simulink subsystem "SiDLEngine"  (R2023b)
settings: Solver=VariableStepAuto  StartTime=0.0  StopTime=10.0  RelTol=1e-3
undefined symbols (not defined in the file): EnvAbsPrs, EnvAirTemp, EnvRair, PlntEngAfrStoich, PlntEngCps, PlntEngGasLhv, PlntEngInTrqLdBpt, PlntEngInTrqSpdBpt, PlntEngNeuralODE, PlntEngSAOpt, PlntEngSIDLNCyl, PlntEngSIDLTimeCETC, PlntEngSIDLTimeCVGT, PlntEngSIDLVd, PlntEngSinj, PlntEngTimeCEGR, PlntEngTimeCIRL, PlntEngTimeCIVL, PlntEngTimeCVCR, PlntEngTimeCWVA
libraries: autolibutils x2, autolibpowerinfoutils x2, autolibhevctrlrcommon x1
settings Model: ModifiedByFormat=The MathWorks, Inc.  Creator=The MathWorks, Inc.  LastModifiedBy=The MathWorks, Inc.
settings SolverCC: MaxZcPerStep=1
settings OptimizationCC: ReuseModelBlockBuffer=off
settings DebuggingCC: UnconnectedInputMsg=warning  UnconnectedOutputMsg=warning  UnconnectedLineMsg=warning
settings ModelReferenceCC: EnableRefExpFcnMdlSchedulingChecks=on
settings RTWCC: DLArmComputeVersion=19.05

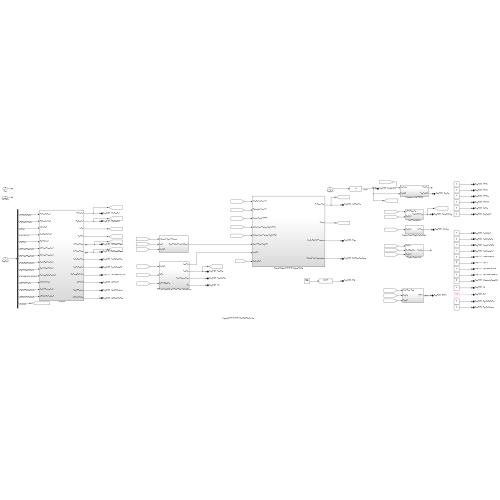
[thumbnail: Simulink's stored preview of the top-level diagram]
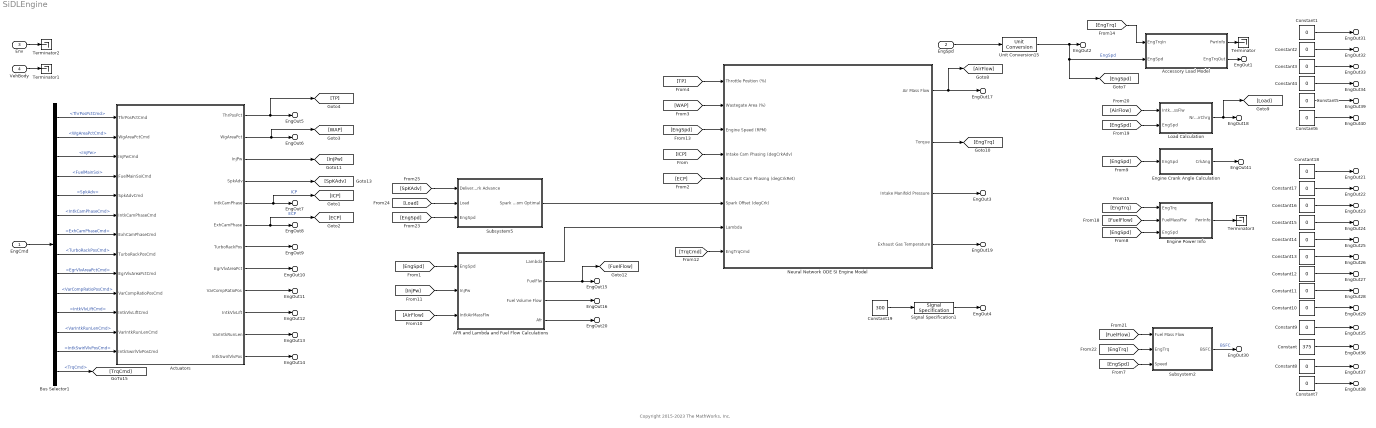
== system SiDLEngine ==
  note: Copyright 2015-2023 The MathWorks, Inc.
  EngCmd : Inport
  EngSpd : Inport  Port=2  Unit=rad/sec
  Env : Inport  Port=3
  VehBody : Inport  Port=4
  AFR and Lambda and Fuel Flow Calculations : Subsystem
  Accessory Load Model : Subsystem
  Actuators : Subsystem
  Bus Selector1 : BusSelector  OutputSignals=ThrPosPctCmd,WgAreaPctCmd,InjPw,FuelMainSoi,SpkAdv,IntkCamPhaseCmd,ExhCamPhaseCmd,TurboRackPosCmd,EgrVlvAreaPctCmd,VarCompRatioPosCmd,IntkVlvLiftCmd,VarIntkRunLenCmd,IntkSwirlVlvPosCmd,TrqCmd
  Constant : Constant  Value=375  SampleTime=-1
  Constant{1..18} (18 alike) : Constant  Value=0  SampleTime=-1
  Constant19 : Constant  Value=300
  Engine Crank Angle Calculation : Subsystem
  Engine Power Info : Subsystem
  Load Calculation : Subsystem
  Neural Network ODE SI Engine Model : Subsystem
  Signal Specification1 : SignalSpecification  Unit=K
  Subsystem2 : Subsystem
  Subsystem5 : Subsystem
  Terminator{,1..3} (4 alike) : Terminator
  Unit Conversion15 : UnitConversion
  EngOut2 : Outport  PortName=EngFdbk  Element=EngSpdOut
  EngOut5 : Outport  PortName=EngFdbk  Element=ThrPosPct
  EngOut6 : Outport  PortName=EngFdbk  Element=WgAreaPct
  EngOut7 : Outport  PortName=EngFdbk  Element=IntkCamPhase
  EngOut8 : Outport  PortName=EngFdbk  Element=ExhCamPhase
  EngOut9 : Outport  PortName=EngFdbk  Element=TurboRackPos
  EngOut10 : Outport  PortName=EngFdbk  Element=EgrVlvAreaPct
  EngOut11 : Outport  PortName=EngFdbk  Element=VarCompRatioPos
  EngOut12 : Outport  PortName=EngFdbk  Element=IntkVlvLift
  EngOut13 : Outport  PortName=EngFdbk  Element=VarIntkRunLen
  EngOut14 : Outport  PortName=EngFdbk  Element=IntkSwirlVlvPos
  EngOut3 : Outport  PortName=EngFdbk  Element=Map
  EngOut4 : Outport  PortName=EngFdbk  Element=Mat
  EngOut15 : Outport  PortName=EngFdbk  Element=FuelFlw
  EngOut16 : Outport  PortName=EngFdbk  Element=FuelVolFlw
  EngOut20 : Outport  PortName=EngFdbk  Element=Afr
  EngOut19 : Outport  PortName=EngFdbk  Element=ExhManGasTemp
  EngOut17 : Outport  PortName=EngFdbk  Element=IntkPortFlw
  EngOut1 : Outport  PortName=EngFdbk  Element=EngTrq
  EngOut18 : Outport  PortName=EngFdbk  Element=NormAirChrg
  EngOut41 : Outport  PortName=EngFdbk  Element=CrkAng
  EngOut30 : Outport  PortName=EngFdbk  Element=BSFC
  EngOut31 : Outport  PortName=EngFdbk  Element=TPHC
  EngOut32 : Outport  PortName=EngFdbk  Element=TPCO
  EngOut33 : Outport  PortName=EngFdbk  Element=TPNOx
  EngOut34 : Outport  PortName=EngFdbk  Element=TPCO2
  EngOut39 : Outport  PortName=EngFdbk  Element=CylPrs
  EngOut40 : Outport  PortName=EngFdbk  Element=EngTrqCrk
  EngOut21 : Outport  PortName=EngFdbk  Element=TurboSpd
  EngOut22 : Outport  PortName=EngFdbk  Element=TurbPrsRatio
  EngOut23 : Outport  PortName=EngFdbk  Element=CompPrsRatio
  EngOut24 : Outport  PortName=EngFdbk  Element=TurbTempOut
  EngOut25 : Outport  PortName=EngFdbk  Element=CompTempOut
  EngOut26 : Outport  PortName=EngFdbk  Element=EgrPct
  EngOut27 : Outport  PortName=EngFdbk  Element=EgrMassFlwRate
  EngOut28 : Outport  PortName=EngFdbk  Element=EgrCoolerTempOut
  EngOut29 : Outport  PortName=EngFdbk  Element=IntercoolerTempOut
  EngOut35 : Outport  PortName=EngFdbk  Element=Iat
  EngOut36 : Outport  PortName=EngFdbk  Element=Ect
  EngOut37 : Outport  PortName=EngFdbk  Element=EgrVlvDeltaPrs
  EngOut38 : Outport  PortName=EngFdbk  Element=EgrVlvInTemp
  wires:
  Actuators/11(VarIntkRunLen) -> EngOut13/1
  Constant12/1 -> EngOut27/1
  Actuators/7(TurboRackPos) -> EngOut9/1
  Actuators/6(ExhCamPhase) -> [ECP], EngOut8/1  "ECP"
  Actuators/9(VarCompRatioPos) -> EngOut11/1
  Constant1/1 -> EngOut31/1
  Engine Crank Angle Calculation/1(CrkAng) -> EngOut41/1
  [EngSpd] -> Engine Crank Angle Calculation/1(EngSpd)
  [EngSpd] -> Engine Power Info/3(EngSpd)
  Subsystem5/1(Spark Retard From Optimal) -> Neural Network ODE SI Engine Model/6(Spark Offset (degCrk))
  Accessory Load Model/2(EngTrqOut) -> EngOut1/1
  [TP] -> Neural Network ODE SI Engine Model/1(Throttle Position (%))
  [ECP] -> Neural Network ODE SI Engine Model/5(Exhaust Cam Phasing (degCrkRet))
  [FuelFlow] -> Engine Power Info/2(FuelMassFlw)
  [EngSpd] -> Neural Network ODE SI Engine Model/3(Engine Speed (RPM))
  Neural Network ODE SI Engine Model/2(Torque) -> [EngTrq]
  [ICP] -> Neural Network ODE SI Engine Model/4(Intake Cam Phasing (degCrkAdv))
  Constant13/1 -> EngOut26/1
  [EngTrq] -> Subsystem2/2(EngTrq)
  Accessory Load Model/1(PwrInfo) -> Terminator/1
  Constant/1 -> EngOut36/1
  Constant10/1 -> EngOut29/1
  Actuators/5(IntkCamPhase) -> [ICP], EngOut7/1  "ICP"
  Neural Network ODE SI Engine Model/3(Intake Manifold Pressure) -> EngOut3/1
  [InjPw] -> AFR and Lambda and Fuel Flow Calculations/2(InjPw)
  Constant8/1 -> EngOut37/1
  Constant4/1 -> EngOut34/1
  Constant15/1 -> EngOut24/1
  [AirFlow] -> AFR and Lambda and Fuel Flow Calculations/3(IntkAirMassFlw)
  Subsystem2/1(BSFC) -> EngOut30/1  "BSFC"
  [EngSpd] -> AFR and Lambda and Fuel Flow Calculations/1(EngSpd)
  [TrqCmd] -> Neural Network ODE SI Engine Model/8(EngTrqCmd)
  [Load] -> Subsystem5/2(Load)
  AFR and Lambda and Fuel Flow Calculations/3(Fuel Volume Flow) -> EngOut16/1
  Actuators/8(EgrVlvAreaPct) -> EngOut10/1
  Constant19/1 -> Signal Specification1/1
  [EngTrq] -> Engine Power Info/1(EngTrq)
  Constant7/1 -> EngOut38/1
  [EngTrq] -> Accessory Load Model/1(EngTrqIn)
  AFR and Lambda and Fuel Flow Calculations/2(FuelFlw) -> [FuelFlow], EngOut15/1
  [EngSpd] -> Load Calculation/2(EngSpd)
  AFR and Lambda and Fuel Flow Calculations/1(Lambda) -> Neural Network ODE SI Engine Model/7(Lambda)
  Neural Network ODE SI Engine Model/1(Air Mass Flow) -> [AirFlow], EngOut17/1
  [AirFlow] -> Load Calculation/1(IntkAirMassFlw)
  Bus Selector1/1 -> Actuators/1(ThrPosPctCmd)  "<ThrPosPctCmd>"
  Constant14/1 -> EngOut25/1
  [EngSpd] -> Subsystem2/3(Speed)
  Constant11/1 -> EngOut28/1
  Constant17/1 -> EngOut22/1
  Actuators/2(WgAreaPct) -> [WAP], EngOut6/1
  AFR and Lambda and Fuel Flow Calculations/4(Afr) -> EngOut20/1
  Constant6/1 -> EngOut40/1
  Constant3/1 -> EngOut33/1
  Neural Network ODE SI Engine Model/4(Exhaust Gas Temperature) -> EngOut19/1
  [EngSpd] -> Subsystem5/3(EngSpd)
  Actuators/10(IntkVlvLift) -> EngOut12/1
  Actuators/4(SpkAdv) -> [SpKAdv]
  Actuators/1(ThrPosPct) -> [TP], EngOut5/1
  Constant16/1 -> EngOut23/1
  [SpKAdv] -> Subsystem5/1(Delivered Spark Advance)
  Engine Power Info/1(PwrInfo) -> Terminator3/1
  Actuators/12(IntkSwirlVlvPos) -> EngOut14/1
  Constant9/1 -> EngOut35/1
  Constant5/1 -> EngOut39/1
  [WAP] -> Neural Network ODE SI Engine Model/2(Wastegate Area (%))
  Actuators/3(InjPw) -> [InjPw]
  [FuelFlow] -> Subsystem2/1(Fuel Mass Flow)
  Constant18/1 -> EngOut21/1
  Load Calculation/1(NrmlzdAirChrg) -> [Load], EngOut18/1
  Constant2/1 -> EngOut32/1
  EngCmd/1 -> Bus Selector1/1
  Bus Selector1/12 -> Actuators/12(VarIntkRunLenCmd)  "<VarIntkRunLenCmd>"
  Bus Selector1/2 -> Actuators/2(WgAreaPctCmd)  "<WgAreaPctCmd>"
  Bus Selector1/6 -> Actuators/6(IntkCamPhaseCmd)  "<IntkCamPhaseCmd>"
  Bus Selector1/11 -> Actuators/11(IntkVlvLiftCmd)  "<IntkVlvLiftCmd>"
  Bus Selector1/3 -> Actuators/3(InjPwCmd)  "<InjPw>"
  Bus Selector1/7 -> Actuators/7(ExhCamPhaseCmd)  "<ExhCamPhaseCmd>"
  Bus Selector1/10 -> Actuators/10(VarCompRatioPosCmd)  "<VarCompRatioPosCmd>"
  Bus Selector1/9 -> Actuators/9(EgrVlvAreaPctCmd)  "<EgrVlvAreaPctCmd>"
  Bus Selector1/13 -> Actuators/13(IntkSwirlVlvPosCmd)  "<IntkSwirlVlvPosCmd>"
  Bus Selector1/14 -> [TrqCmd]  "<TrqCmd>"
  Bus Selector1/5 -> Actuators/5(SpkAdvCmd)  "<SpkAdv>"
  Bus Selector1/8 -> Actuators/8(TurboRackPosCmd)  "<TurboRackPosCmd>"
  Bus Selector1/4 -> Actuators/4(FuelMainSoiCmd)  "<FuelMainSoi>"
  EngSpd/1 -> Unit Conversion15/1
  Unit Conversion15/1 -> Accessory Load Model/2(EngSpd), [EngSpd], EngOut2/1  "EngSpd"
  VehBody/1 -> Terminator1/1
  Env/1 -> Terminator2/1
  Signal Specification1/1 -> EngOut4/1

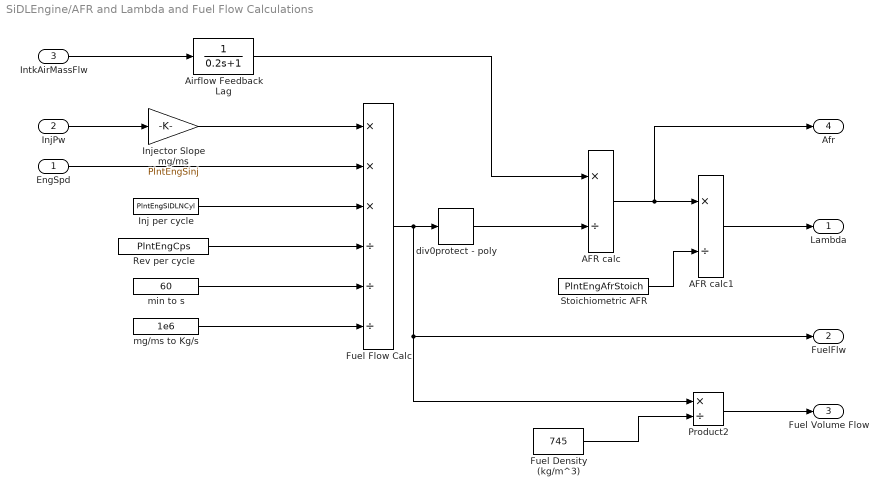
== system SiDLEngine/AFR and Lambda and Fuel Flow Calculations ==
  EngSpd : Inport
  InjPw : Inport  Port=2
  IntkAirMassFlw : Inport  Port=3
  AFR calc : Product  Inputs=*/
  AFR calc1 : Product  Inputs=*/
  Airflow Feedback Lag : TransferFcn  Denominator=[0.2 1]
  Fuel Density (kg/m^3) : Constant  Value=745
  Fuel Flow Calc : Product  Inputs=***///
  Inj per cycle : Constant  Value=PlntEngSIDLNCyl
  Injector Slope mg/ms : Gain  Gain=PlntEngSinj
  Product2 : Product  Inputs=*/
  Rev per cycle : Constant  Value=PlntEngCps
  Stoichiometric AFR : Constant  Value=PlntEngAfrStoich
  div0protect - poly : autolibutils/div0protect - poly  thresh=1e-6  ZeroCross1=off  aMode=aMode
  mg/ms to Kg/s : Constant  Value=1e6
  min to s : Constant  Value=60
  Lambda : Outport  VectorParamsAs1DForOutWhenUnconnected=off
  FuelFlw : Outport  Port=2  VectorParamsAs1DForOutWhenUnconnected=off
  Fuel Volume Flow : Outport  Port=3
  Afr : Outport  Port=4  VectorParamsAs1DForOutWhenUnconnected=off
  wires:
  Fuel Flow Calc/1 -> div0protect - poly/1, Product2/1, FuelFlw/1
  Fuel Density (kg/m^3)/1 -> Product2/2
  Product2/1 -> Fuel Volume Flow/1
  AFR calc1/1 -> Lambda/1
  IntkAirMassFlw/1 -> Airflow Feedback Lag/1
  EngSpd/1 -> Fuel Flow Calc/2
  Inj per cycle/1 -> Fuel Flow Calc/3
  Injector Slope mg/ms/1 -> Fuel Flow Calc/1
  mg/ms to Kg/s/1 -> Fuel Flow Calc/6
  min to s/1 -> Fuel Flow Calc/5
  Stoichiometric AFR/1 -> AFR calc1/2
  div0protect - poly/1 -> AFR calc/2
  InjPw/1 -> Injector Slope mg/ms/1
  AFR calc/1 -> AFR calc1/1, Afr/1
  Rev per cycle/1 -> Fuel Flow Calc/4
  Airflow Feedback Lag/1 -> AFR calc/1

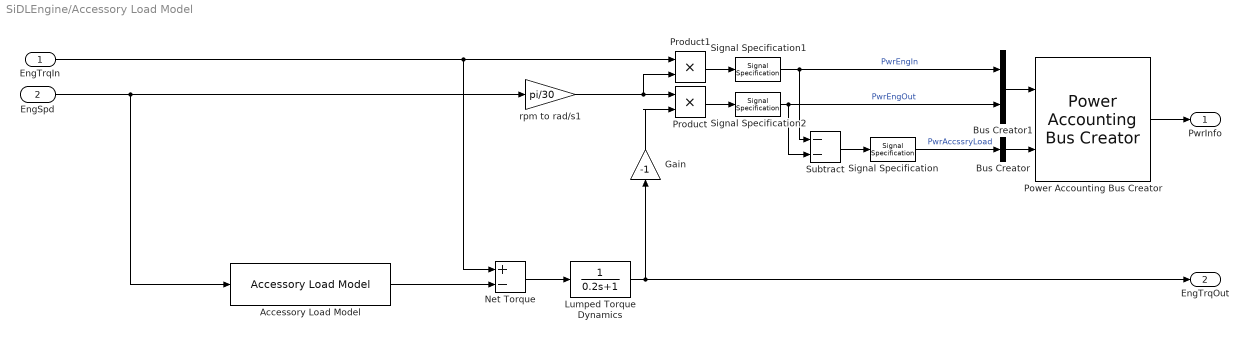
== system SiDLEngine/Accessory Load Model ==
  EngTrqIn : Inport
  EngSpd : Inport  Port=2
  Accessory Load Model : autolibhevctrlrcommon/Accessory Load Model  AccPwrTbl=PlntEngSIDLAccPwrTbl  AccSpdBpts=PlntEngSIDLAccSpdBpt
  Bus Creator : BusCreator  Inputs=1
  Bus Creator1 : BusCreator  Inputs=2
  Gain : Gain  Gain=-1
  Lumped Torque Dynamics : TransferFcn  Denominator=[0.2 1]
  Net Torque : Sum  Inputs=+-
  Power Accounting Bus Creator : autolibpowerinfoutils/Power Accounting Bus Creator  AssctBlkSelPopup=Parent  RefBlkName='libraryname/blkname'  PwrTrnsfrdCheckBox=on  PwrNotTrnsfrdCheckBox=on  PwrStoredCheckBox=off  aMode=aMode
  Product : Product
  Product1 : Product
  Signal Specification : SignalSpecification  Unit=W
  Signal Specification1 : SignalSpecification  Unit=W
  Signal Specification2 : SignalSpecification  Unit=W
  Subtract : Sum  Inputs=--
  rpm to rad/s1 : Gain  Gain=pi/30
  PwrInfo : Outport  VectorParamsAs1DForOutWhenUnconnected=off
  EngTrqOut : Outport  Port=2  Unit=N*m  VectorParamsAs1DForOutWhenUnconnected=off
  wires:
  Gain/1 -> Product/2
  Signal Specification2/1 -> Bus Creator1/2, Subtract/2  "PwrEngOut"
  Signal Specification1/1 -> Bus Creator1/1, Subtract/1  "PwrEngIn"
  rpm to rad/s1/1 -> Product/1, Product1/2
  Product1/1 -> Signal Specification1/1
  Product/1 -> Signal Specification2/1
  Power Accounting Bus Creator/1 -> PwrInfo/1
  Signal Specification/1 -> Bus Creator/1  "PwrAccssryLoad"
  Subtract/1 -> Signal Specification/1
  EngTrqIn/1 -> Net Torque/1, Product1/1
  Bus Creator1/1 -> Power Accounting Bus Creator/1
  Bus Creator/1 -> Power Accounting Bus Creator/2
  Net Torque/1 -> Lumped Torque Dynamics/1
  Lumped Torque Dynamics/1 -> Gain/1, EngTrqOut/1
  EngSpd/1 -> rpm to rad/s1/1, Accessory Load Model/1
  Accessory Load Model/1 -> Net Torque/2

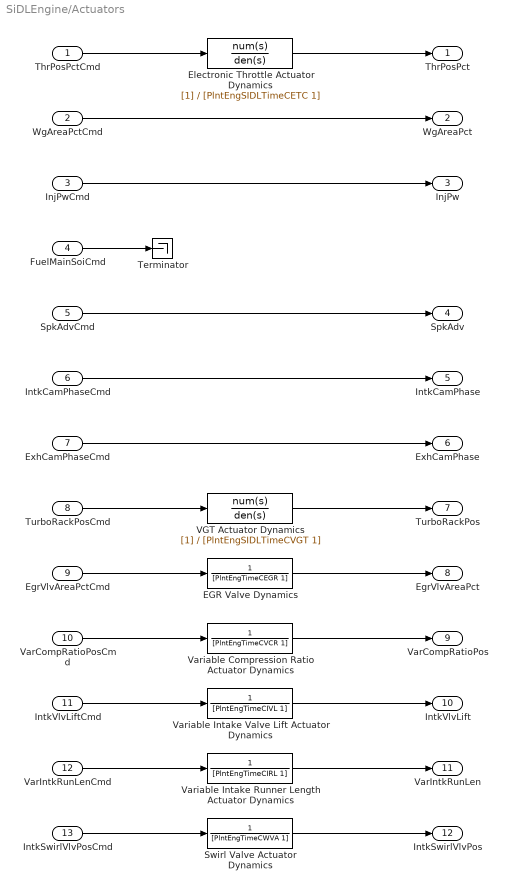
== system SiDLEngine/Actuators ==
  ThrPosPctCmd : Inport  Unit=%
  WgAreaPctCmd : Inport  Port=2  Unit=%
  InjPwCmd : Inport  Port=3  Unit=ms
  FuelMainSoiCmd : Inport  Port=4  Unit=deg
  SpkAdvCmd : Inport  Port=5  Unit=deg
  IntkCamPhaseCmd : Inport  Port=6  Unit=deg
  ExhCamPhaseCmd : Inport  Port=7  Unit=deg
  TurboRackPosCmd : Inport  Port=8  Unit=1
  EgrVlvAreaPctCmd : Inport  Port=9  Unit=%
  VarCompRatioPosCmd : Inport  Port=10
  IntkVlvLiftCmd : Inport  Port=11
  VarIntkRunLenCmd : Inport  Port=12
  IntkSwirlVlvPosCmd : Inport  Port=13
  EGR Valve Dynamics : TransferFcn  Denominator=[PlntEngTimeCEGR 1]
  Electronic Throttle Actuator Dynamics : TransferFcn  Denominator=[PlntEngSIDLTimeCETC 1]
  Swirl Valve Actuator Dynamics : TransferFcn  Denominator=[PlntEngTimeCWVA 1]
  Terminator : Terminator
  VGT Actuator Dynamics : TransferFcn  Denominator=[PlntEngSIDLTimeCVGT 1]
  Variable Compression Ratio Actuator Dynamics : TransferFcn  Denominator=[PlntEngTimeCVCR 1]
  Variable Intake Runner Length Actuator Dynamics : TransferFcn  Denominator=[PlntEngTimeCIRL 1]
  Variable Intake Valve Lift Actuator Dynamics : TransferFcn  Denominator=[PlntEngTimeCIVL 1]
  ThrPosPct : Outport  Unit=%  VectorParamsAs1DForOutWhenUnconnected=off
  WgAreaPct : Outport  Port=2  Unit=%  VectorParamsAs1DForOutWhenUnconnected=off
  InjPw : Outport  Port=3  VectorParamsAs1DForOutWhenUnconnected=off
  SpkAdv : Outport  Port=4  VectorParamsAs1DForOutWhenUnconnected=off
  IntkCamPhase : Outport  Port=5  Unit=deg  VectorParamsAs1DForOutWhenUnconnected=off
  ExhCamPhase : Outport  Port=6  Unit=deg  VectorParamsAs1DForOutWhenUnconnected=off
  TurboRackPos : Outport  Port=7  Unit=1  VectorParamsAs1DForOutWhenUnconnected=off
  EgrVlvAreaPct : Outport  Port=8  Unit=%  VectorParamsAs1DForOutWhenUnconnected=off
  VarCompRatioPos : Outport  Port=9  VectorParamsAs1DForOutWhenUnconnected=off
  IntkVlvLift : Outport  Port=10  VectorParamsAs1DForOutWhenUnconnected=off
  VarIntkRunLen : Outport  Port=11  VectorParamsAs1DForOutWhenUnconnected=off
  IntkSwirlVlvPos : Outport  Port=12  VectorParamsAs1DForOutWhenUnconnected=off
  wires:
  SpkAdvCmd/1 -> SpkAdv/1
  EgrVlvAreaPctCmd/1 -> EGR Valve Dynamics/1
  TurboRackPosCmd/1 -> VGT Actuator Dynamics/1
  EGR Valve Dynamics/1 -> EgrVlvAreaPct/1
  VGT Actuator Dynamics/1 -> TurboRackPos/1
  InjPwCmd/1 -> InjPw/1
  VarIntkRunLenCmd/1 -> Variable Intake Runner Length Actuator Dynamics/1
  VarCompRatioPosCmd/1 -> Variable Compression Ratio Actuator Dynamics/1
  ThrPosPctCmd/1 -> Electronic Throttle Actuator Dynamics/1
  IntkSwirlVlvPosCmd/1 -> Swirl Valve Actuator Dynamics/1
  IntkVlvLiftCmd/1 -> Variable Intake Valve Lift Actuator Dynamics/1
  FuelMainSoiCmd/1 -> Terminator/1
  Electronic Throttle Actuator Dynamics/1 -> ThrPosPct/1
  WgAreaPctCmd/1 -> WgAreaPct/1
  ExhCamPhaseCmd/1 -> ExhCamPhase/1
  IntkCamPhaseCmd/1 -> IntkCamPhase/1
  Swirl Valve Actuator Dynamics/1 -> IntkSwirlVlvPos/1
  Variable Intake Runner Length Actuator Dynamics/1 -> VarIntkRunLen/1
  Variable Intake Valve Lift Actuator Dynamics/1 -> IntkVlvLift/1
  Variable Compression Ratio Actuator Dynamics/1 -> VarCompRatioPos/1

== system SiDLEngine/Engine Crank Angle Calculation ==
  EngSpd : Inport  Unit=rev/min
  Integrator : Integrator  UpperSaturationLimit=720  LowerSaturationLimit=0  WrapState=on  WrappedStateUpperValue=360*PlntEngCps  WrappedStateLowerValue=0
  RPM to deg/s : Gain  Gain=180/30
  CrkAng : Outport  Unit=deg  VectorParamsAs1DForOutWhenUnconnected=off
  wires:
  Integrator/1 -> CrkAng/1
  EngSpd/1 -> RPM to deg/s/1
  RPM to deg/s/1 -> Integrator/1

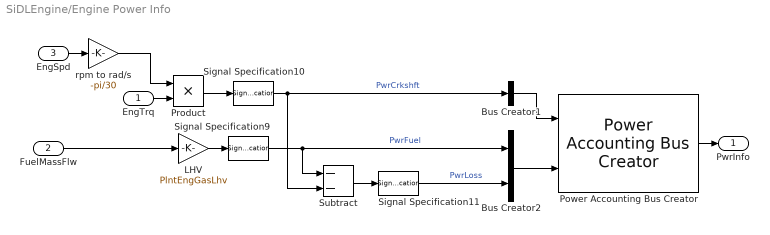
== system SiDLEngine/Engine Power Info ==
  EngTrq : Inport
  FuelMassFlw : Inport  Port=2
  EngSpd : Inport  Port=3
  Bus Creator1 : BusCreator  Inputs=1
  Bus Creator2 : BusCreator  Inputs=2
  LHV : Gain  Gain=PlntEngGasLhv
  Power Accounting Bus Creator : autolibpowerinfoutils/Power Accounting Bus Creator  AssctBlkSelPopup=Parent  RefBlkName='autolibsharedmappedengines/Mapped SI Engine'  PwrTrnsfrdCheckBox=on  PwrNotTrnsfrdCheckBox=on  PwrStoredCheckBox=off  aMode=aMode
  Product : Product
  Signal Specification10 : SignalSpecification  Unit=W
  Signal Specification11 : SignalSpecification  Unit=W
  Signal Specification9 : SignalSpecification  Unit=W
  Subtract : Sum  Inputs=--
  rpm to rad/s : Gain  Gain=-pi/30
  PwrInfo : Outport  VectorParamsAs1DForOutWhenUnconnected=off
  wires:
  Signal Specification9/1 -> Subtract/1, Bus Creator2/1  "PwrFuel"
  Signal Specification10/1 -> Bus Creator1/1, Subtract/2  "PwrCrkshft"
  Bus Creator2/1 -> Power Accounting Bus Creator/2
  Product/1 -> Signal Specification10/1
  Signal Specification11/1 -> Bus Creator2/2  "PwrLoss"
  Subtract/1 -> Signal Specification11/1
  EngSpd/1 -> rpm to rad/s/1
  rpm to rad/s/1 -> Product/1
  LHV/1 -> Signal Specification9/1
  Bus Creator1/1 -> Power Accounting Bus Creator/1
  FuelMassFlw/1 -> LHV/1
  Power Accounting Bus Creator/1 -> PwrInfo/1
  EngTrq/1 -> Product/2

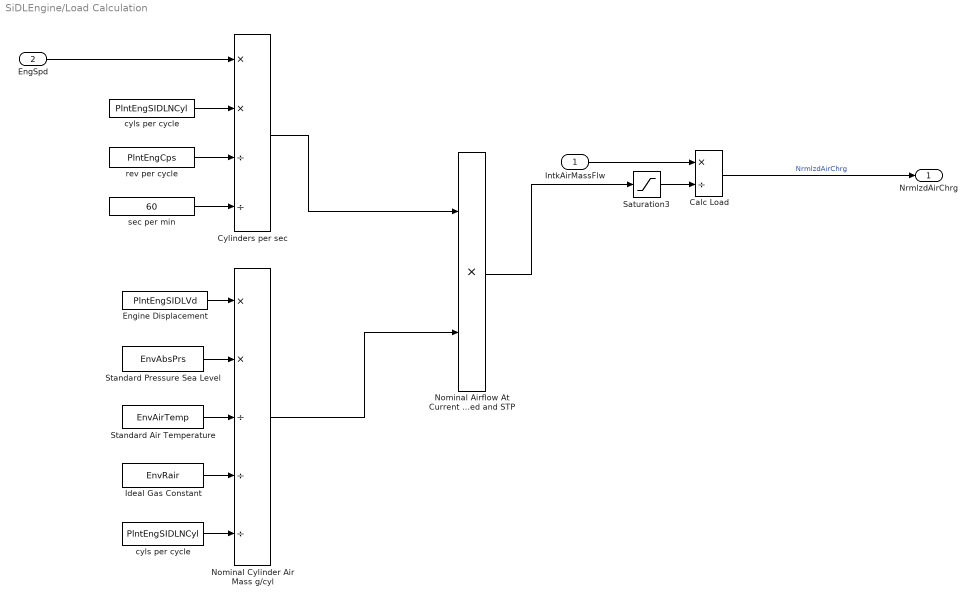
== system SiDLEngine/Load Calculation ==
  IntkAirMassFlw : Inport  Unit=kg/s
  EngSpd : Inport  Port=2  Unit=rev/min
  Calc Load : Product  Inputs=*/
  Cylinders per sec : Product  Inputs=**//  RndMeth=Zero
  Engine Displacement : Constant  Value=PlntEngSIDLVd
  Ideal Gas Constant : Constant  Value=EnvRair
  Nominal Airflow At Current Speed and STP : Product  Inputs=**  RndMeth=Zero
  Nominal Cylinder Air Mass g/cyl : Product  Inputs=**///  RndMeth=Zero
  Saturation3 : Saturate  UpperLimit=1e6  LowerLimit=0.0001  ZeroCross=off
  Standard Air Temperature : Constant  Value=EnvAirTemp
  Standard Pressure Sea Level : Constant  Value=EnvAbsPrs
  cyls per cycle : Constant  Value=PlntEngSIDLNCyl
  "cyls per cycle " : Constant  Value=PlntEngSIDLNCyl
  rev per cycle : Constant  Value=PlntEngCps
  sec per min : Constant  Value=60
  NrmlzdAirChrg : Outport  Unit=1  VectorParamsAs1DForOutWhenUnconnected=off
  wires:
  "cyls per cycle "/1 -> Nominal Cylinder Air Mass g/cyl/5
  Saturation3/1 -> Calc Load/2
  sec per min/1 -> Cylinders per sec/4
  Cylinders per sec/1 -> Nominal Airflow At Current Speed and STP/1
  EngSpd/1 -> Cylinders per sec/1
  Nominal Airflow At Current Speed and STP/1 -> Saturation3/1
  Nominal Cylinder Air Mass g/cyl/1 -> Nominal Airflow At Current Speed and STP/2
  rev per cycle/1 -> Cylinders per sec/3
  Ideal Gas Constant/1 -> Nominal Cylinder Air Mass g/cyl/4
  Standard Pressure Sea Level/1 -> Nominal Cylinder Air Mass g/cyl/2
  Engine Displacement/1 -> Nominal Cylinder Air Mass g/cyl/1
  Standard Air Temperature/1 -> Nominal Cylinder Air Mass g/cyl/3
  cyls per cycle/1 -> Cylinders per sec/2
  IntkAirMassFlw/1 -> Calc Load/1
  Calc Load/1 -> NrmlzdAirChrg/1  "NrmlzdAirChrg"

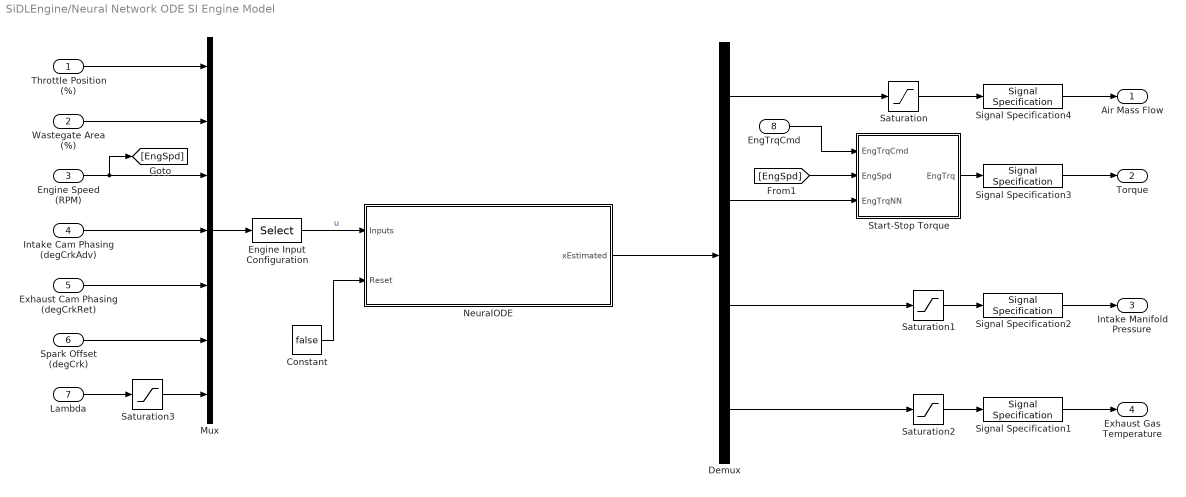
== system SiDLEngine/Neural Network ODE SI Engine Model ==
  Throttle Position (%) : Inport
  Wastegate Area (%) : Inport  Port=2
  Engine Speed (RPM) : Inport  Port=3
  Intake Cam Phasing (degCrkAdv) : Inport  Port=4
  Exhaust Cam Phasing (degCrkRet) : Inport  Port=5
  Spark Offset (degCrk) : Inport  Port=6
  Lambda : Inport  Port=7
  EngTrqCmd : Inport  Port=8
  Constant : Constant  Value=false
  Demux : Demux
  Engine Input Configuration : Selector  InputPortWidth=7  IndexOptions=Index vector (dialog)  Indices=PlntEngSIDLEngineType  OutputSizes=1
  Mux : Mux  Inputs=7
  NeuralODE : Subsystem  mask(Neural ODE model){inferenceModel=Custom block, model=PlntEngNeuralODE, x0=PlntEngNeuralODE.data.Y0, muU=PlntEngNeuralODE.data.muU, sigU=PlntEngNeuralODE.data.sigU, muY=PlntEngNeuralODE.data.muY, sigY=PlntEngNeuralODE.data.sigY}
      mask prompts: inferenceModel "Inference model used"; model "Trained model parameters (struct)"; x0 "Initial state of the integrator"; muU "Input data mean value"; sigU "Input data standard deviation"; muY "Output data mean value"; sigY "Output data standard deviation"
      mask help: This block calculates a Neural ODE model for simulation
      mask init:
      | nin = model.data.nin;
      |     nout = model.data.nout;
      |     inputDelays = model.trainingOptions.inputDelays;
      |     outputDelays = model.trainingOptions.outputDelays;
      |     
      |     % nu is used in the Simulink model
      |     nu = nin*(inputDelays(end)+1);
      |     
      |     inputDelays = 0; % make sure we use 0
      |     
      |     % State augmentation switch,to properly setup the outputs size
      |     if model.trainingOptions.useAugmentation
      |         selectedIndices = 1:nout;
      |         % augment x0
      |         x0 = [x0;zeros(model.trainingOptions.augmentationSize,1)];
      |         stateVectorSize = size(x0,1);
      |     else
      |         selectedIndices = 1:nout;    
      |         stateVectorSize = size(x0,1);
      |     end
      mask TypeOptions inferenceModel: Predict block (requires Deep Learning Toolbox) | Custom block
      mask DialogControl ParameterGroupVar Prompt: Model Parameters
      mask DialogControl Container3 Prompt: Data standardization (z-score)
  Saturation : Saturate  UpperLimit=Inf  LowerLimit=0  ZeroCross=off
  Saturation1 : Saturate  UpperLimit=2.3e5  LowerLimit=10000  ZeroCross=off
  Saturation2 : Saturate  UpperLimit=Inf  LowerLimit=300  ZeroCross=off
  Saturation3 : Saturate  UpperLimit=1  LowerLimit=0.7  ZeroCross=off
  Signal Specification1 : SignalSpecification  Unit=K
  Signal Specification2 : SignalSpecification  Unit=Pa
  Signal Specification3 : SignalSpecification  Unit=N*m
  Signal Specification4 : SignalSpecification  Unit=kg/s
  Start-Stop Torque : Subsystem
  Air Mass Flow : Outport
  Torque : Outport  Port=2
  Intake Manifold Pressure : Outport  Port=3
  Exhaust Gas Temperature : Outport  Port=4
  wires:
  Saturation3/1 -> Mux/7
  Demux/1 -> Saturation/1
  Throttle Position (%)/1 -> Mux/1
  Start-Stop Torque/1(EngTrq) -> Signal Specification3/1
  Demux/2 -> Start-Stop Torque/3(EngTrqNN)
  [EngSpd] -> Start-Stop Torque/2(EngSpd)
  EngTrqCmd/1 -> Start-Stop Torque/1(EngTrqCmd)
  Saturation2/1 -> Signal Specification1/1
  Saturation1/1 -> Signal Specification2/1
  Saturation/1 -> Signal Specification4/1
  Signal Specification4/1 -> Air Mass Flow/1
  Signal Specification3/1 -> Torque/1
  Signal Specification2/1 -> Intake Manifold Pressure/1
  Signal Specification1/1 -> Exhaust Gas Temperature/1
  Demux/4 -> Saturation2/1
  Demux/3 -> Saturation1/1
  Engine Speed (RPM)/1 -> Mux/3, [EngSpd]
  Spark Offset (degCrk)/1 -> Mux/6
  Exhaust Cam Phasing (degCrkRet)/1 -> Mux/5
  Wastegate Area (%)/1 -> Mux/2
  Lambda/1 -> Saturation3/1
  Intake Cam Phasing (degCrkAdv)/1 -> Mux/4
  NeuralODE/1(xEstimated) -> Demux/1
  Mux/1 -> Engine Input Configuration/1
  Constant/1 -> NeuralODE/2(Reset)
  Engine Input Configuration/1 -> NeuralODE/1(Inputs)  "u"

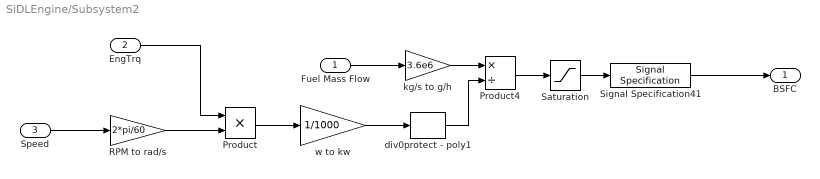
== system SiDLEngine/Subsystem2 ==
  Fuel Mass Flow : Inport
  EngTrq : Inport  Port=2
  Speed : Inport  Port=3
  Product : Product
  Product4 : Product  Inputs=*/
  RPM to rad/s : Gain  Gain=2*pi/60
  Saturation : Saturate  UpperLimit=500  LowerLimit=0  ZeroCross=off
  Signal Specification41 : SignalSpecification  Unit=g/(kW*hr)
  div0protect - poly1 : autolibutils/div0protect - poly  thresh=0.01  ZeroCross1=off  aMode=aMode
  kg/s to g/h : Gain  Gain=3.6e6
  w to kw : Gain  Gain=1/1000
  BSFC : Outport
  wires:
  Signal Specification41/1 -> BSFC/1
  Fuel Mass Flow/1 -> kg/s to g/h/1
  Speed/1 -> RPM to rad/s/1
  Saturation/1 -> Signal Specification41/1
  EngTrq/1 -> Product/1
  Product/1 -> w to kw/1
  Product4/1 -> Saturation/1
  div0protect - poly1/1 -> Product4/2
  kg/s to g/h/1 -> Product4/1
  RPM to rad/s/1 -> Product/2
  w to kw/1 -> div0protect - poly1/1

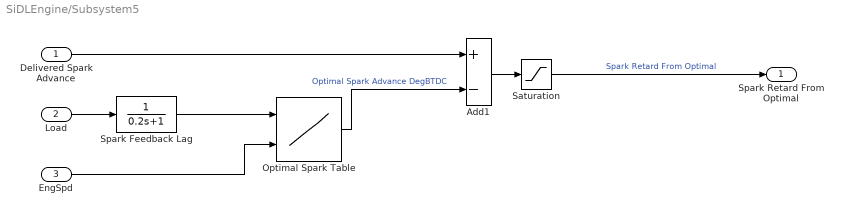
== system SiDLEngine/Subsystem5 ==
  Delivered Spark Advance : Inport
  Load : Inport  Port=2
  EngSpd : Inport  Port=3
  Add1 : Sum  Inputs=+-
  Optimal Spark Table : Lookup_n-D  LookupTableObject=''  BreakpointsForDimension1=PlntEngInTrqLdBpt  BreakpointsForDimension2=PlntEngInTrqSpdBpt  Table=PlntEngSAOpt  ExtrapMethod=Clip  InternalRulePriority=Speed  RndMeth=Simplest
      settings: InputPortMap=u0,u1
  Saturation : Saturate  UpperLimit=0  LowerLimit=-10
  Spark Feedback Lag : TransferFcn  Denominator=[0.2 1]
  Spark Retard From Optimal : Outport
  wires:
  Add1/1 -> Saturation/1
  Load/1 -> Spark Feedback Lag/1
  Saturation/1 -> Spark Retard From Optimal/1  "Spark Retard From Optimal"
  EngSpd/1 -> Optimal Spark Table/2
  Optimal Spark Table/1 -> Add1/2  "Optimal Spark Advance DegBTDC"
  Delivered Spark Advance/1 -> Add1/1
  Spark Feedback Lag/1 -> Optimal Spark Table/1

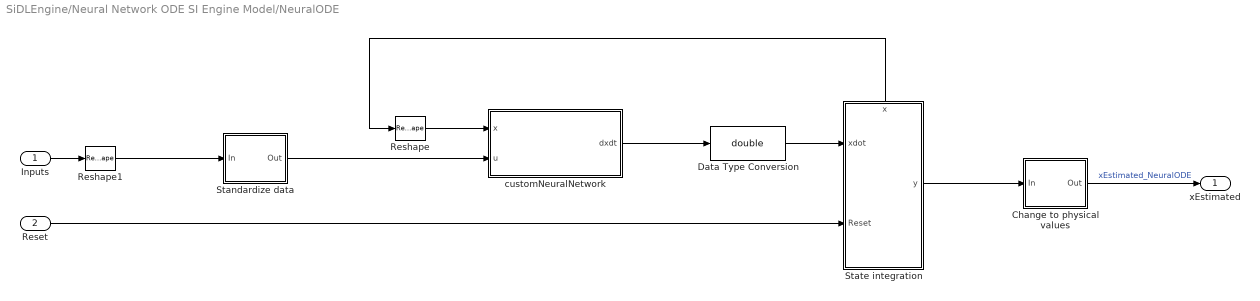
== system SiDLEngine/Neural Network ODE SI Engine Model/NeuralODE ==
  Inputs : Inport
  Reset : Inport  Port=2
  Change to physical values : Subsystem  mask{mu=muY, sig=sigY}
      mask prompts: mu "Mean value"; sig "Standard deviation"
  Data Type Conversion : DataTypeConversion  OutDataTypeStr=double  SaturateOnIntegerOverflow=off  RndMeth=Floor
  Reshape : Reshape  OutputDimensionality=Column vector (2-D)
  Reshape1 : Reshape  OutputDimensionality=Column vector (2-D)
  Standardize data : Subsystem  mask{mu=muU, sig=sigU}
      mask prompts: mu "Mean value"; sig "Standard deviation"
  State integration : Subsystem  TreatAsAtomicUnit=on
      settings: PortSchema="{\"entries\":[{\"content\":{\"sides\":[{\"content\":{\"connectorIds\":[\"In1\",\"In2\"]},\"type\":\"ConnectorPlacement.EquallySpacedRectSide\",\"uuid\":\"3e2d00db-1226-4178-8dae-e6ef3bd536db\"},{\"content\":{\"connectorIds\":[\"Out1\"],\"side\":\"RIGHT\"},\"type\":\"ConnectorPlacement.EquallySpacedRectSide\",\"uuid\":\"79e8d3d4-b743-4294-9854-667dc210d77c\"},{\"content\":{\"connectorIds\":[\"Out2\"],\"side\":\"TOP\"},\"type\":\"ConnectorPlacement.EquallySpacedRectSide\",\"uuid\":\"81266a48-5ba2-4b71-8bcc-751f191337ce\"}]},\"type\":\"ConnectorPlacement.EquallySpacedConnector\",\"uuid\":\"38953849-82ad-438f-bb50-56898b24f709\"}],\"packageUris\":[\"http://schema.mathworks.com/mf0/Connector/R2020b\"],\"version\":\"1.0\"}"
  customNeuralNetwork : Subsystem  VariantControl=Custom block
  xEstimated : Outport
  wires:
  Reset/1 -> State integration/2(Reset)
  customNeuralNetwork/1(dxdt) -> Data Type Conversion/1
  State integration/2(x) -> Reshape/1
  State integration/1(y) -> Change to physical values/1(In)
  Reshape/1 -> customNeuralNetwork/1(x)
  Inputs/1 -> Reshape1/1
  Change to physical values/1(Out) -> xEstimated/1  "xEstimated_NeuralODE"
  Standardize data/1(Out) -> customNeuralNetwork/2(u)
  Reshape1/1 -> Standardize data/1(In)
  Data Type Conversion/1 -> State integration/1(xdot)

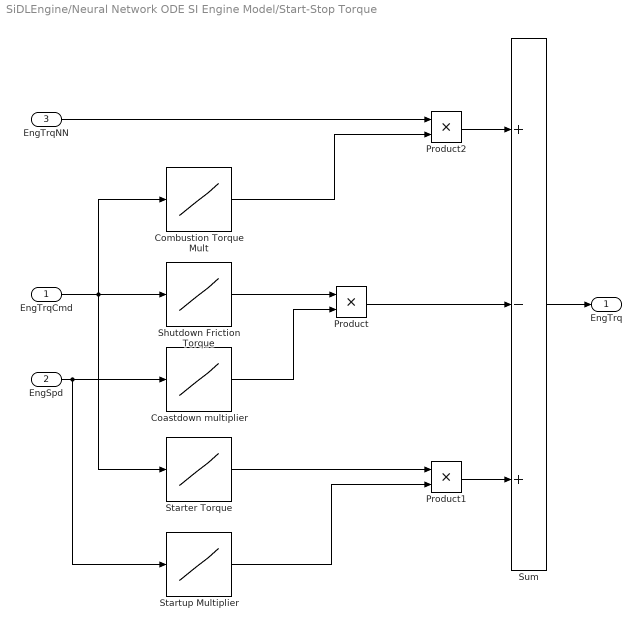
== system SiDLEngine/Neural Network ODE SI Engine Model/Start-Stop Torque ==
  EngTrqCmd : Inport
  EngSpd : Inport  Port=2
  EngTrqNN : Inport  Port=3
  Coastdown multiplier : Lookup_n-D  NumberOfTableDimensions=1  BreakpointsForDimension1=[-1 0 500]  Table=[-1 0 1]  ExtrapMethod=Clip  InternalRulePriority=Speed  RndMeth=Simplest
  Combustion Torque Mult : Lookup_n-D  NumberOfTableDimensions=1  BreakpointsForDimension1=[0 1e-2]  Table=[0 1]  ExtrapMethod=Clip  InternalRulePriority=Speed  RndMeth=Simplest
  Product : Product
  Product1 : Product
  Product2 : Product
  Shutdown Friction Torque : Lookup_n-D  NumberOfTableDimensions=1  BreakpointsForDimension1=[0 1e-6]  Table=[10 0]  ExtrapMethod=Clip  InternalRulePriority=Speed  RndMeth=Simplest
  Starter Torque : Lookup_n-D  NumberOfTableDimensions=1  BreakpointsForDimension1=[0 1e-6]  Table=[0 20]  ExtrapMethod=Clip  InternalRulePriority=Speed  RndMeth=Simplest
  Startup Multiplier : Lookup_n-D  NumberOfTableDimensions=1  BreakpointsForDimension1=[0 500]  Table=[1 0]  ExtrapMethod=Clip  InternalRulePriority=Speed  RndMeth=Simplest
  Sum : Sum  Inputs=+-+
  EngTrq : Outport
  wires:
  Combustion Torque Mult/1 -> Product2/2
  Product2/1 -> Sum/1
  Product1/1 -> Sum/3
  Startup Multiplier/1 -> Product1/2
  Starter Torque/1 -> Product1/1
  EngSpd/1 -> Coastdown multiplier/1, Startup Multiplier/1
  Coastdown multiplier/1 -> Product/2
  Sum/1 -> EngTrq/1
  EngTrqNN/1 -> Product2/1
  Product/1 -> Sum/2
  Shutdown Friction Torque/1 -> Product/1
  EngTrqCmd/1 -> Shutdown Friction Torque/1, Starter Torque/1, Combustion Torque Mult/1

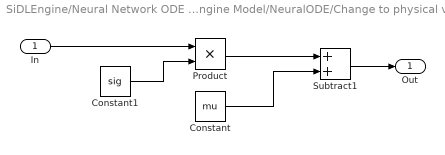
== system SiDLEngine/Neural Network ODE SI Engine Model/NeuralODE/Change to physical values ==
  In : Inport
  Constant : Constant  Value=mu
  Constant1 : Constant  Value=sig
  Product : Product
  Subtract1 : Sum
  Out : Outport
  wires:
  In/1 -> Product/1
  Subtract1/1 -> Out/1
  Constant/1 -> Subtract1/2
  Product/1 -> Subtract1/1
  Constant1/1 -> Product/2

== system SiDLEngine/Neural Network ODE SI Engine Model/NeuralODE/Standardize data ==
  In : Inport
  Constant : Constant  Value=mu
  Constant1 : Constant  Value=sig
  Divide : Product  Inputs=*/
  Subtract1 : Sum  Inputs=+-
  Out : Outport
  wires:
  Constant/1 -> Subtract1/2
  In/1 -> Subtract1/1
  Subtract1/1 -> Divide/1
  Divide/1 -> Out/1
  Constant1/1 -> Divide/2

== system SiDLEngine/Neural Network ODE SI Engine Model/NeuralODE/State integration ==
  xdot : Inport
  Reset : Inport  Port=2
  Continuous-Time Integrator : Subsystem  VariantControl=Continuous
  output selector : Selector  InputPortWidth=stateVectorSize  IndexOptions=Index vector (dialog)  Indices=selectedIndices  OutputSizes=1
      settings: AttributesFormatString=|
      | InputSize: %<InputPortWidth>
      | Selected: %<Indices>
  y : Outport
  x : Outport  Port=2
  wires:
  Reset/1 -> Continuous-Time Integrator/2(Reset)
  Continuous-Time Integrator/1(Out1) -> x/1, output selector/1
  output selector/1 -> y/1
  xdot/1 -> Continuous-Time Integrator/1(xdot)

== system SiDLEngine/Neural Network ODE SI Engine Model/NeuralODE/customNeuralNetwork ==
  x : Inport
  u : Inport  Port=2
  customNeuralNetwork : MATLAB Function  TreatAsAtomicUnit=on  VariantControl=customNeuralNetwork  mask{netParams_double=model.model}
      mask prompts: netParams_double "Model parameters (struct of double())"
  dxdt : Outport
  wires:
  x/1 -> customNeuralNetwork/1(x)
  customNeuralNetwork/1(dxdt) -> dxdt/1
  u/1 -> customNeuralNetwork/2(u)

== system SiDLEngine/Neural Network ODE SI Engine Model/NeuralODE/State integration/Continuous-Time Integrator ==
  xdot : Inport
  Reset : Inport  Port=2
  Constant : Constant  Value=x0
  Continuous-Time Integrator : Integrator  ExternalReset=either  InitialConditionSource=external  InitialCondition=[x0;zeros(size(x0,1),1)]
  Out1 : Outport
  wires:
  Reset/1 -> Continuous-Time Integrator/2
  Constant/1 -> Continuous-Time Integrator/3
  Continuous-Time Integrator/1 -> Out1/1
  xdot/1 -> Continuous-Time Integrator/1

== matlab function SiDLEngine/Neural Network ODE SI Engine Model/NeuralODE/customNeuralNetwork/customNeuralNetwork ==
  data: x input; u input; netParams_double parameter; dxdt output
function dxdt = NeuralODE(x, u, netParams_double)

%#codegen

dxdt = autoblkssidleval(x,u,netParams_double);
